simulink model "CarHalf_Verif_Lin"  (R2021b)
settings: Solver=VariableStepAuto  StartTime=0.0  StopTime=10.0  RelTol=1e-3
settings Model: Creator=reece  LastModifiedBy=reece

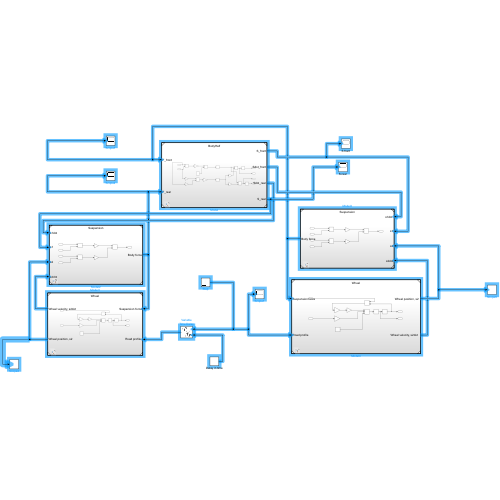
[thumbnail: Simulink's stored preview of the top-level diagram]
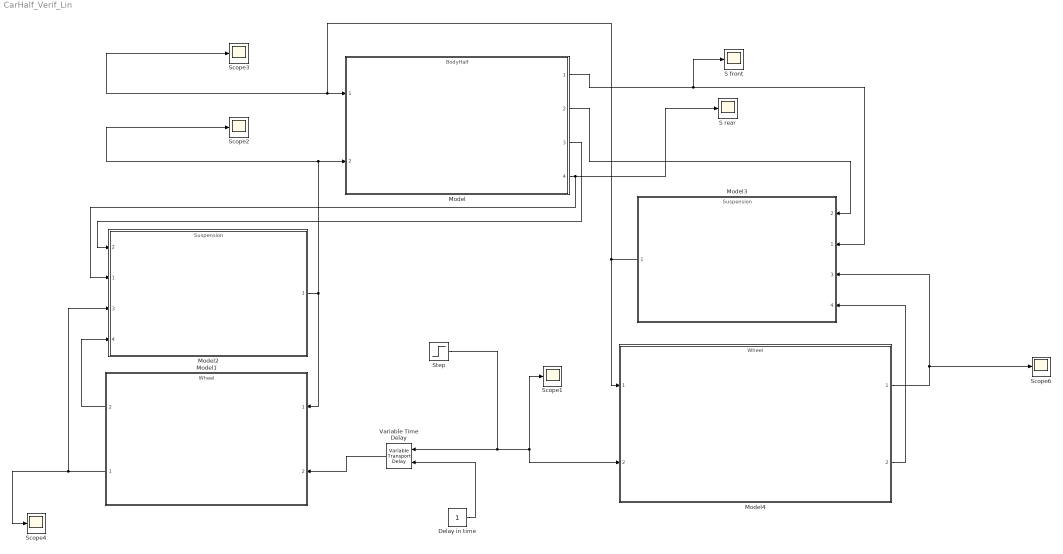
== system CarHalf_Verif_Lin ==
  Delay in time : Constant
  Model : ModelReference  ModelNameDialog=BodyHalf.slx  SimulationMode=Normal  ModelReferenceVersion=7.0
  Model1 : ModelReference  ModelNameDialog=Wheel.slx  SimulationMode=Normal  ModelReferenceVersion=1.11
      settings: PortSchema="{\"entries\":[{\"content\":{\"sides\":[{\"content\":{\"connectorIds\":[\"In1\",\"In2\"]},\"type\":\"ConnectorPlacement.EquallySpacedRectSide\",\"uuid\":\"71a4e87f-1851-4422-8936-4b87f85412fd\"},{\"content\":{\"connectorIds\":[\"Out2\",\"Out1\"],\"side\":\"RIGHT\"},\"type\":\"ConnectorPlacement.EquallySpacedRectSide\",\"uuid\":\"a8cbb71a-0d58-4894-b904-4ecd4e9fe1a2\"},{\"content\":{\"connectorIds\":[],\"side\":\"TOP\"},\"type\":\"ConnectorPlacement.EquallySpacedRectSide\",\"uuid\":\"1c77120d-7330-4516-954d-d61049980f4f\"}]},\"type\":\"ConnectorPlacement.EquallySpacedConnector\",\"uuid\":\"3f64bc7a-ba11-44ce-9e66-88e335d5dfb1\"}],\"packageUris\":[\"http://schema.mathworks.com/mf0/Connector/R2020b\"],\"version\":\"1.0\"}"
  Model2 : ModelReference  ModelNameDialog=Suspension.slx  SimulationMode=Normal  ModelReferenceVersion=1.8
      settings: PortSchema="{\"entries\":[{\"content\":{\"sides\":[{\"content\":{\"connectorIds\":[\"In2\",\"In1\",\"In3\",\"In4\"]},\"type\":\"ConnectorPlacement.EquallySpacedRectSide\",\"uuid\":\"94601151-747d-4428-9167-f5fe05b2d5ec\"},{\"content\":{\"connectorIds\":[\"Out1\"],\"side\":\"RIGHT\"},\"type\":\"ConnectorPlacement.EquallySpacedRectSide\",\"uuid\":\"dff19792-31ea-4015-87a5-b27b5b8418bd\"},{\"content\":{\"connectorIds\":[],\"side\":\"TOP\"},\"type\":\"ConnectorPlacement.EquallySpacedRectSide\",\"uuid\":\"ecb08bd5-caa0-4733-8680-fe03693d318b\"}]},\"type\":\"ConnectorPlacement.EquallySpacedConnector\",\"uuid\":\"5a835372-3a50-49f7-b808-dc60be46a96a\"}],\"packageUris\":[\"http://schema.mathworks.com/mf0/Connector/R2020b\"],\"version\":\"1.0\"}"
  Model3 : ModelReference  ModelNameDialog=Suspension.slx  SimulationMode=Normal  ModelReferenceVersion=1.8
      settings: PortSchema="{\"entries\":[{\"content\":{\"sides\":[{\"content\":{\"connectorIds\":[\"In2\",\"In1\",\"In3\",\"In4\"]},\"type\":\"ConnectorPlacement.EquallySpacedRectSide\",\"uuid\":\"94601151-747d-4428-9167-f5fe05b2d5ec\"},{\"content\":{\"connectorIds\":[\"Out1\"],\"side\":\"RIGHT\"},\"type\":\"ConnectorPlacement.EquallySpacedRectSide\",\"uuid\":\"dff19792-31ea-4015-87a5-b27b5b8418bd\"},{\"content\":{\"connectorIds\":[],\"side\":\"TOP\"},\"type\":\"ConnectorPlacement.EquallySpacedRectSide\",\"uuid\":\"ecb08bd5-caa0-4733-8680-fe03693d318b\"}]},\"type\":\"ConnectorPlacement.EquallySpacedConnector\",\"uuid\":\"5a835372-3a50-49f7-b808-dc60be46a96a\"}],\"packageUris\":[\"http://schema.mathworks.com/mf0/Connector/R2020b\"],\"version\":\"1.0\"}"
  Model4 : ModelReference  ModelNameDialog=Wheel.slx  SimulationMode=Normal  ModelReferenceVersion=1.11
  S front : Scope
  S rear : Scope
  Scope{1..4,6} (5 alike) : Scope
  Step : Step  SampleTime=0
  Variable Time Delay : VariableTransportDelay  MaximumDelay=10
  wires:
  Model4/1 -> Scope6/1, Model3/3
  Step/1 -> Variable Time Delay/1, Scope1/1, Model4/2
  Model/3 -> Model2/2
  Model/2 -> Model3/2
  Model/1 -> Model3/1, S front/1
  Variable Time Delay/1 -> Model1/2
  Model1/2 -> Model2/4
  Model2/1 -> Model1/1, Model/2, Scope2/1
  Model3/1 -> Model4/1, Scope3/1, Model/1
  Model4/2 -> Model3/4
  Delay in time/1 -> Variable Time Delay/2
  Model/4 -> S rear/1, Model2/1
  Model1/1 -> Scope4/1, Model2/3
